simulink model "BLDC_PWM_control"  (R2024b)
settings: Solver=odeN  StartTime=0.0  StopTime=35  MaxStep=Ts_motor  RelTol=1e-3  EnableMultiTasking=on
InitFcn:
  | load bldcData
model workspace (MAT data in the model file):
  encoderResolution = 2000
  hallOffset = '0.5'
  indexOffset = 850
  polePairs = '4'
undefined symbols (not defined in the file): DiscIntNeverNeededParam, Ts_motor
libraries: nesl_utility x14, fl_lib x9, ee_lib x7, spsPWMGeneratorDCDCLib x1, slpidlib x1, simulink x1
settings Model: SimulationMode=accelerator  Creator=The MathWorks, Inc.
settings SolverCC: AlgebraicLoopSolver=TrustRegion  AutoInsertRateTranBlk=on
settings DataIOCC: LimitDataPoints=on  SaveFormat=Array  SaveOutput=off  SaveTime=off  ReturnWorkspaceOutputs=off
settings OptimizationCC: DefaultParameterBehavior=Inlined  OptimizeBlockIOStorage=off  BufferReuse=off  GlobalBufferReuse=off  ExpressionFolding=off  ExpressionDepthLimit=2147483647  LocalBlockOutputs=off  ZeroExternalMemoryAtStartup=off  InitFltsAndDblsToZero=on  NoFixptDivByZeroProtection=on  EfficientFloat2IntCast=on  EfficientMapNaN2IntZero=off  LifeSpan=Inf  MaxStackSize=64  OptimizeDataStoreBuffers=off  BusAssignmentInplaceUpdate=off  EfficientTunableParamExpr=on
settings DebuggingCC: ReadBeforeWriteMsg=DisableAll  WriteAfterWriteMsg=DisableAll  WriteAfterReadMsg=DisableAll  CheckSSInitialOutputMsg=off  SignalResolutionControl=TryResolveAllWithWarning  SolverPrmCheckMsg=warning  InheritedTsInSrcMsg=none  MultiTaskDSMMsg=none  MultiTaskCondExecSysMsg=none  TasksWithSamePriorityMsg=none  SigSpecEnsureSampleTimeMsg=none  IntegerOverflowMsg=none  ParameterPrecisionLossMsg=none  FcnCallInpInsideContextMsg=warning  UnconnectedInputMsg=warning  UnconnectedOutputMsg=warning  UnconnectedLineMsg=warning  AllowSymbolicDim=off  StateNameClashWarn=warning  PregeneratedLibrarySubsystemCodeDiagnostic=none  SFUnexpectedBacktrackingDiag=warning  SFNoUnconditionalDefaultTransitionDiag=warning  SFExecutionAtInitializationDiag=none  IntegerSaturationMsg=none  ArithmeticOperatorsInVariantConditions=warning
settings HardwareCC: ProdBitPerChar=16  ProdBitPerInt=16  ProdBitPerPointer=32  ProdBitPerSizeT=32  ProdBitPerPtrDiffT=32  ProdLargestAtomicInteger=Integer  ProdLargestAtomicFloat=None  ProdWordSize=16  ProdLongLongMode=on  ProdHWDeviceType=Texas Instruments->C2000  TargetBitPerChar=16  TargetBitPerInt=16  TargetBitPerPointer=16  TargetLargestAtomicInteger=Integer  TargetIntDivRoundTo=Zero  TargetEndianess=LittleEndian  TargetWordSize=16  TargetHWDeviceType=TI C2000
settings ModelReferenceCC: EnableRefExpFcnMdlSchedulingChecks=on  PropagateSignalLabelsOutOfModel=off
settings SFSimCC: SimUseLocalCustomCode=off  MATLABDynamicMemAlloc=off
settings RTWCC: Description=Embedded Coder  SystemTargetFile=ert.tlc  TemplateMakefile=ert_default_tmf  GenerateReport=on  RTWUseLocalCustomCode=off  Toolchain=Texas Instruments Code Composer Studio (C2000)  IncludeHyperlinkInReport=on  LaunchReport=on  GenerateTraceInfo=on  GenerateTraceReport=on  GenerateTraceReportSl=on  GenerateTraceReportSf=on  GenerateTraceReportEml=on  GPUComputeCapability=3.5
settings CodeAppCC: IgnoreCustomStorageClasses=off  CustomSymbolStrType=$N$R$M  StateflowObjectComments=on  InternalIdentifier=Classic
settings ERTTargetCC: MultiwordLength=2048  InlinedParameterPlacement=Hierarchical  ERTCustomFileTemplate=example_file_process.tlc  ConvertIfToSwitch=off  SuppressUnreachableDefaultCases=off  MemSecPackage=tic2000demospkg  DynamicArrayContainerType=coder::array
settings ConfigComp: CovMetricSettings=dw  CovSaveCumulativeToWorkspaceVar=on  CovSaveSingleToWorkspaceVar=on  CovExternalEMLEnable=off  CovSFcnEnable=off

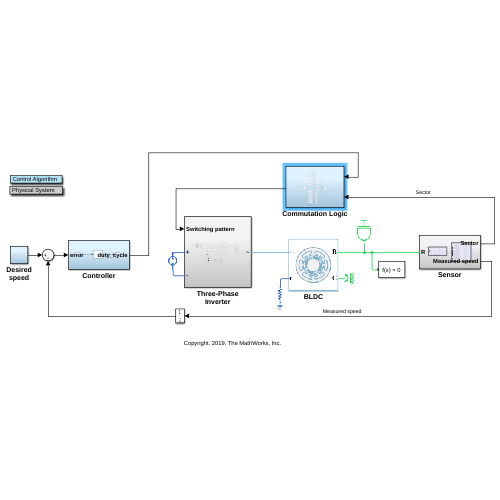
[thumbnail: Simulink's stored preview of the top-level diagram]
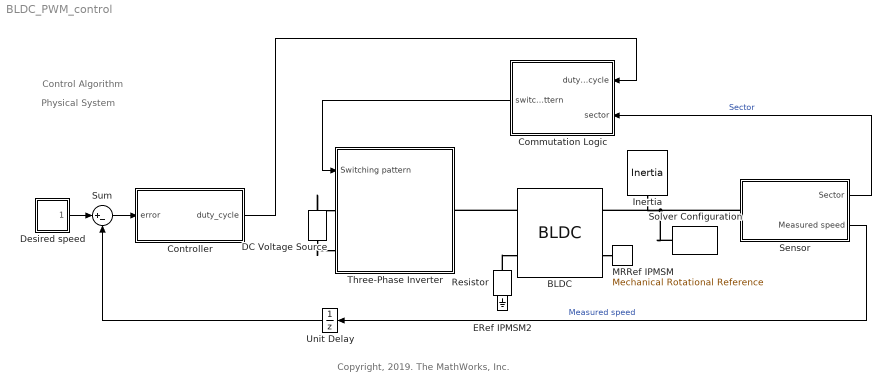
== system BLDC_PWM_control ==
  note: Copyright, 2019. The MathWorks, Inc.
  note: Control Algorithm
  note: Physical System
  BLDC : ee_lib/Electromechanical/Permanent Magnet/BLDC  port_option=ee.enum.threePhasePort.composite  rotor_param=1  pm_flux_linkage=0.18 Wb  theta_constant=120/4 deg  emf_max=9.6 V  w_meas=600 rpm  DphiDtheta_tab=[0, -.1528, -.1528, .1528, .1528, 0] Wb/rad  back_emf_tab=[0, -9.6, -9.6, 9.6, 9.6, 0] V  rotor_angle_tab=[0, 7.5, 22.5, 37.5, 52.5, 60] deg  nPolePairs=4  axes_param=1  winding_type=ee.enum.statorconnection.wye  stator_param=ee.enum.statorparam.LdLqL0  machine_param=ee.enum.dqparameterization.constant  Ld=0.0001 H  Lq=0.0001 H  idVec=[-200, 0, 200] A  iqVec=[-200, 0, 200] A  LdMatrix=0.00022 * ones(3, 3) H  LqMatrix=0.00022 * ones(3, 3) H  L0=0.00016 H  Ls=0.0002 H  Lm=0 H  Ms=0.00002 H  Rs=0.001 Ohm  zero_sequence=ee.enum.park.zerosequence.include  loss_param=ee.enum.ironloss.none  losses_oc=[0, 0, 0] W  losses_sc=[0, 0, 0] W  f_losses=60 Hz  Isc_losses=95 A  J=0 kg*m^2  lam=0.1 N*m/(rad/s)  i_d_specify=off  i_d_priority=None  i_d=0 A  i_d_nominal_specify=off  i_d_nominal_value=1  i_d_nominal_unit=A  i_q_specify=off  i_q_priority=None  i_q=0 A  i_q_nominal_specify=off  i_q_nominal_value=1  i_q_nominal_unit=A  torque_specify=off  torque_priority=None  torque=0 N*m  torque_nominal_specify=off  torque_nominal_value=1  torque_nominal_unit=N*m  angular_velocity_specify=off  angular_velocity_priority=High  angular_velocity=0 rpm  angular_velocity_nominal_specify=off  angular_velocity_nominal_value=1  angular_velocity_nominal_unit=rpm  angular_position_specify=off  angular_position_priority=High  angular_position=0 deg  angular_position_nominal_specify=off  angular_position_nominal_value=1  angular_position_nominal_unit=deg  alpha=3.93e-3 1/K  alpha_flux=-0.001 1/K  Tmeas=298.15 K  stator_thermal_mass=100 J/K  rotor_thermal_mass=200 J/K  Rm_percent_rotor=90  Rd_percent_rotor=30  temperatureA_specify=off  temperatureA_priority=High  temperatureA=25 degC  temperatureA_nominal_specify=off  temperatureA_nominal_value=1  temperatureA_nominal_unit=degC  temperatureB_specify=off  temperatureB_priority=High  temperatureB=25 degC  temperatureB_nominal_specify=off  temperatureB_nominal_value=1  temperatureB_nominal_unit=degC  temperatureC_specify=off  temperatureC_priority=High  temperatureC=25 degC  temperatureC_nominal_specify=off  temperatureC_nominal_value=1  temperatureC_nominal_unit=degC  temperatureR_specify=off  temperatureR_priority=High  temperatureR=25 degC  temperatureR_nominal_specify=off  temperatureR_nominal_value=1  temperatureR_nominal_unit=degC
      settings: InternalSimscapePortConfiguration="{\"Bottom\":[],\"Left\":[{\"id\":\"N\",\"label\":\"~\",\"type\":\"foundation.electrical.three_phase\"},{\"id\":\"n\",\"label\":\"n\",\"type\":\"foundation.electrical.electrical\"}],\"Right\":[{\"id\":\"R\",\"label\":\"R\",\"type\":\"foundation.mechanical.rotational.rotational\"},{\"id\":\"C\",\"label\":\"C\",\"type\":\"foundation.mechanical.rotational.rotational\"}],\"Top\":[]}"
  Commutation Logic : Subsystem
  Controller : Subsystem
  DC Voltage Source : ee_lib/Additional Components/SPICE Sources/DC Voltage Source  DC=500 V
  Desired speed : Subsystem
  ERef IPMSM2 : fl_lib/Electrical/Electrical Elements/Electrical Reference
  Inertia : fl_lib/Mechanical/Rotational Elements/Inertia  inertia=2 kg*m^2  num_ports=foundation.enum.numPorts2.one  w_specify=off  w_priority=High  w=0 rpm  w_nominal_specify=off  w_nominal_value=1  w_nominal_unit=rad/s  t_specify=off  t_priority=High  t=0 N*m  t_nominal_specify=off  t_nominal_value=1  t_nominal_unit=N*m
  MRRef IPMSM : fl_lib/Mechanical/Rotational Elements/Mechanical Rotational Reference
  Resistor : fl_lib/Electrical/Electrical Elements/Resistor  R=1e9 Ohm  i_specify=off  i_priority=None  i=0 A  i_nominal_specify=off  i_nominal_value=1  i_nominal_unit=A  v_specify=off  v_priority=None  v=0 V  v_nominal_specify=off  v_nominal_value=1  v_nominal_unit=V
  Sensor : Subsystem
  Solver Configuration : nesl_utility/Solver Configuration  PhysicalDomain=network_engine_domain  SubClassName=solver  LeftPortType=input  RightPortType=generic  Tones=[]  Harmonics=[]  SimulateNoise=off  Profile=off  UseLocalSampling=off  EnableSwitchedLinearOptims=on  FrequencyDomain=off  UseCCode=off  RelTol=0.001  AbsTol=1e-06  MinStep=1e-09  ToWorkspace=off  RevertToSquareIcSolve=off  NumHomotopyIterations=100  PhasorMode=off  PhasorModeNumHarmonics=1  ConsistencySolver=NEWTON_FTOL  IndexReductionMethod=DerivativeReplacement  DoDC=off  ResidualTolerance=1e-09  ConsistencyTolSource=GLOBAL  ConsistencyAbsTol=0.001  ConsistencyRelTol=0.001  ConsistencyTolFactor=0.001  UseLocalSolver=on  LocalSolverChoice=NE_BACKWARD_EULER_ADVANCER  ResolveIndetEquations=on  FunctionEvalNumThread=1  LocalSolverSampleTime=Ts_motor  DoFixedCost=on  MaxNonlinIter=2  MaxModeIter=2  ComputeImpulses=off  ImpulseIterations=2  LinearAlgebra=auto  LinearAlgebraNumThread=0  EquationFormulation=NE_TIME_EF  DelaysMemoryBudget=1024  AutomaticFiltering=on  FilteringTimeConstant=0.001  PartitionStorageMethod=AS_NEEDED  PartitionMemoryBudget=1024  PartitionMethod=FAST  MultibodyUseLocalSolver=off  MultibodyLocalSolverChoice=ODE1  MultibodyLocalSolverSampleTime=0.001
  Sum : Sum  Inputs=|+-
  Three-Phase Inverter : Subsystem
  Unit Delay : UnitDelay  SampleTime=-1  HasFrameUpgradeWarning=on
  wires:
  Sensor/1(Sector) -> Commutation Logic/2(sector)  "Sector"
  Sum/1 -> Controller/1(error)
  Unit Delay/1 -> Sum/2
  Desired speed/1(Out1) -> Sum/1
  Sensor/2(Measured speed) -> Unit Delay/1  "Measured speed"
  Commutation Logic/1("  switching_pattern") -> Three-Phase Inverter/1(Switching pattern)
  Controller/1(duty_cycle) -> Commutation Logic/1(duty_cycle)
  connections:
  BLDC/RConn2 -- MRRef IPMSM/LConn1
  Sensor/LConn1 -- Inertia/LConn1 -- BLDC/RConn1 -- Solver Configuration/RConn1
  Resistor/LConn1 -- BLDC/LConn2
  ERef IPMSM2/LConn1 -- Resistor/RConn1
  DC Voltage Source/LConn1 -- Three-Phase Inverter/LConn1
  DC Voltage Source/RConn1 -- Three-Phase Inverter/LConn2
  BLDC/LConn1 -- Three-Phase Inverter/RConn1

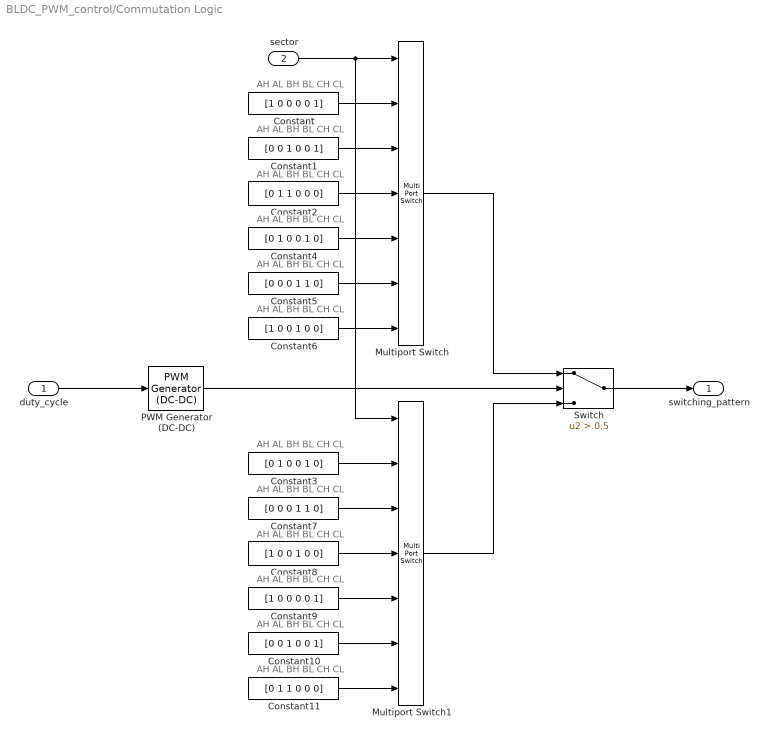
== system BLDC_PWM_control/Commutation Logic ==
  note: AH AL BH BL CH CL
  note: AH AL BH BL CH CL
  note: AH AL BH BL CH CL
  note: AH AL BH BL CH CL
  note: AH AL BH BL CH CL
  note: AH AL BH BL CH CL
  note: AH AL BH BL CH CL
  note: AH AL BH BL CH CL
  note: AH AL BH BL CH CL
  note: AH AL BH BL CH CL
  note: AH AL BH BL CH CL
  note: AH AL BH BL CH CL
  duty_cycle : Inport
  sector : Inport  Port=2
  Constant : Constant  Value=[1 0 0 0 0 1]
  Constant1 : Constant  Value=[0 0 1 0 0 1]
  Constant10 : Constant  Value=[0 0 1 0 0 1]
  Constant11 : Constant  Value=[0 1 1 0 0 0]
  Constant2 : Constant  Value=[0 1 1 0 0 0]
  Constant3 : Constant  Value=[0 1 0 0 1 0]
  Constant4 : Constant  Value=[0 1 0 0 1 0]
  Constant5 : Constant  Value=[0 0 0 1 1 0]
  Constant6 : Constant  Value=[1 0 0 1 0 0]
  Constant7 : Constant  Value=[0 0 0 1 1 0]
  Constant8 : Constant  Value=[1 0 0 1 0 0]
  Constant9 : Constant  Value=[1 0 0 0 0 1]
  Multiport Switch : MultiPortSwitch  Inputs=6  SaturateOnIntegerOverflow=off  InputSameDT=off
  Multiport Switch1 : MultiPortSwitch  Inputs=6  SaturateOnIntegerOverflow=off  InputSameDT=off
  PWM Generator (DC-DC) : spsPWMGeneratorDCDCLib/PWM Generator (DC-DC)  Fsw=1000  Ts=Ts_motor
  Switch : Switch  Criteria=u2 > Threshold  Threshold=0.5  SaturateOnIntegerOverflow=off  InputSameDT=off
  "  switching_pattern" : Outport  VectorParamsAs1DForOutWhenUnconnected=off
  wires:
  Constant6/1 -> Multiport Switch/7
  Constant4/1 -> Multiport Switch/5
  sector/1 -> Multiport Switch1/1, Multiport Switch/1
  Constant1/1 -> Multiport Switch/3
  Constant2/1 -> Multiport Switch/4
  Constant5/1 -> Multiport Switch/6
  Constant/1 -> Multiport Switch/2
  Constant9/1 -> Multiport Switch1/5
  Constant11/1 -> Multiport Switch1/7
  Constant3/1 -> Multiport Switch1/2
  Constant7/1 -> Multiport Switch1/3
  Constant10/1 -> Multiport Switch1/6
  Constant8/1 -> Multiport Switch1/4
  PWM Generator (DC-DC)/1 -> Switch/2
  Switch/1 -> "  switching_pattern"/1
  Multiport Switch/1 -> Switch/1
  Multiport Switch1/1 -> Switch/3
  duty_cycle/1 -> PWM Generator (DC-DC)/1

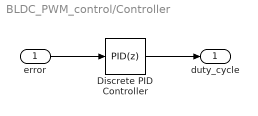
== system BLDC_PWM_control/Controller ==
  error : Inport
  Discrete PID Controller : slpidlib/PID Controller  Controller=PID  Form=Parallel  TimeDomain=Discrete-time  UseExternalTs=off  SampleTime=Ts_motor  IntegratorMethod=Forward Euler  FilterMethod=Forward Euler  ControllerParametersSource=internal  P=0.01  I=0.1  UseKiTs=off  D=0  UseExternalDerivativeSource=off  N=100  UseFilter=on  TunerSelectOption=Transfer Function Based (PID Tuner App)  InitialConditionSource=internal  InitialConditionForIntegrator=0  InitialConditionForFilter=0  DifferentiatorICPrevScaledInput=0  ExternalReset=none  TrackingMode=off  Kt=1  LimitOutput=on  SatLimitsSource=internal  UpperSaturationLimit=1  LowerSaturationLimit=0.5  LinearizeAsGain=off  AntiWindupMode=back-calculation  Kb=1  LimitIntegrator=off  UpperIntegratorSaturationLimit=inf  LowerIntegratorSaturationLimit=-inf  POutMin=[]  POutMax=[]  IOutMin=[]  IOutMax=[]  DOutMin=[]  DOutMax=[]  NOutMin=[]  NOutMax=[]  SumOutMin=[]  SumOutMax=[]  SaturationOutMin=[]  SaturationOutMax=[]  PParamMin=[]  PParamMax=[]  IParamMin=[]  IParamMax=[]  DParamMin=[]  DParamMax=[]  NParamMin=[]  NParamMax=[]  KbParamMin=[]  KbParamMax=[]  KtParamMin=[]  KtParamMax=[]  KbOutMin=[]  KbOutMax=[]  KtOutMin=[]  KtOutMax=[]  IntegratorOutMin=[]  IntegratorOutMax=[]  FilterOutMin=[]  FilterOutMax=[]  SumI1OutMin=[]  SumI1OutMax=[]  SumI2OutMin=[]  SumI2OutMax=[]  SumI3OutMin=[]  SumI3OutMax=[]  SumI4OutMin=[]  SumI4OutMax=[]  SumDOutMin=[]  SumDOutMax=[]  DifferentiatorOutMin=[]  DifferentiatorOutMax=[]  FilterDiffOutCoefMin=[]  FilterDiffOutCoefMax=[]  ReciprocalOutMin=[]  ReciprocalOutMax=[]  SumDenOutMin=[]  SumDenOutMax=[]  SumNumOutMin=[]  SumNumOutMax=[]  DivideOutMin=[]  DivideOutMax=[]  UdiffTsProdOutMin=[]  UdiffTsProdOutMax=[]  NTsProdOutMin=[]  NTsProdOutMax=[]  UintegralTsProdOutMin=[]  UintegralTsProdOutMax=[]  UngainTsProdOutMin=[]  UngainTsProdOutMax=[]  ClampingZeroOutDataTypeStr=Inherit: Inherit via back propagation  ClampingZeroOutMin=[]  ClampingZeroOutMax=[]  FilterDenConstantOutDataTypeStr=Inherit: Inherit via back propagation  FilterDenConstantOutMin=[]  FilterDenConstantOutMax=[]  PCopyOutDataTypeStr=Inherit: Inherit via back propagation  PCopyOutMin=[]  PCopyOutMax=[]  NCopyOutDataTypeStr=Inherit: Inherit via back propagation  NCopyOutMin=[]  NCopyOutMax=[]  IntegratorContinuousStateAttributes=''  IntegratorStateMustResolveToSignalObject=off  IntegratorRTWStateStorageClass=Auto  FilterContinuousStateAttributes=''  FilterStateMustResolveToSignalObject=off  FilterRTWStateStorageClass=Auto  ParallelPVariant=InternalParameters  IdealPVariant=Disabled  IVariant=InternalParameters  DVariant=InternalParameters  IntegratorVariant=Discrete  SatVariant=Enabled  AWVariant=BackCalculation  PCopyVariant=Disabled  TRVariant=Disabled  FdbkBlocksVariant=Forward  IdealPFdbkVariant=Disabled  SatFdbkVariant=Disabled  DerivativeFilterVariant=ForwardEulerFilter  NVariant=InternalParameters  NCopyVariant=Disabled  FilterICVariant=InternalICsFilter  IntegratorICVariant=InternalICs  ExternalResetVariant=Disabled  TRSumVariant=Passthrough  SumFdbkVariant=Disabled  SumVariant=Sum_PID  TsampFilterVariant=InternalTs  TsampNgainVariant=Passthrough  TsampIntegralVariant=Disabled_SignalSpec  ExternalSaturationOutDataTypeStr=Inherit: Same as second input  DerivativeSourceVariant=ErrorSignal  PreIntVariant=InternalPreInt
  duty_cycle : Outport
  wires:
  Discrete PID Controller/1 -> duty_cycle/1
  error/1 -> Discrete PID Controller/1

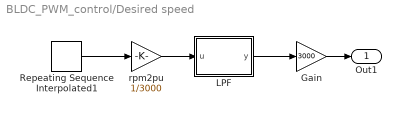
== system BLDC_PWM_control/Desired speed ==
  Gain : Gain  Gain=3000
  LPF : Subsystem
  Repeating Sequence Interpolated1 : simulink/Sources/Repeating Sequence Interpolated  OutValues=[0 1025/2 1025/2 1025 1025 2050 2050 2050]  TimeValues=[0 10 20 30 40 50 60 70]/2  LookUpMeth=Interpolation-Use End Values  tsamp=Ts_motor  OutMin=[]  OutMax=[]  OutDataTypeStr=double  OutputDataTypeScalingMode=double  OutDataType=fixdt(0,8)  OutScaling=2^-10
  rpm2pu : Gain  Gain=1/3000  RndMeth=Simplest  OutDataTypeStr=Inherit: Same as input
  Out1 : Outport
  wires:
  rpm2pu/1 -> LPF/1(u)
  Repeating Sequence Interpolated1/1 -> rpm2pu/1
  LPF/1(y) -> Gain/1
  Gain/1 -> Out1/1

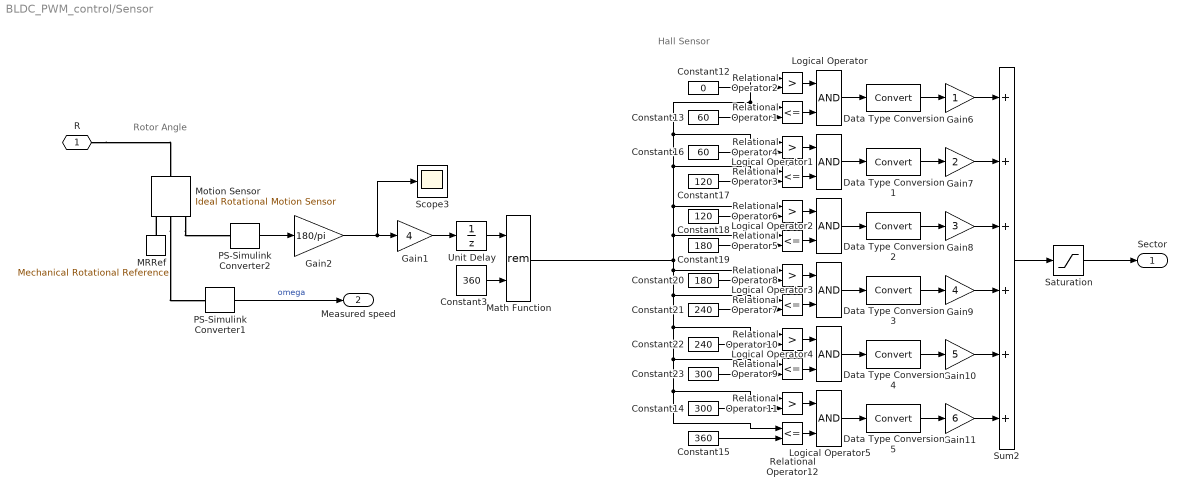
== system BLDC_PWM_control/Sensor ==
  note: Rotor Angle
  note: Hall Sensor
  Constant12 : Constant  Value=0
  Constant13 : Constant  Value=60
  Constant14 : Constant  Value=300
  Constant15 : Constant  Value=360
  Constant16 : Constant  Value=60
  Constant17 : Constant  Value=120
  Constant18 : Constant  Value=120
  Constant19 : Constant  Value=180
  Constant20 : Constant  Value=180
  Constant21 : Constant  Value=240
  Constant22 : Constant  Value=240
  Constant23 : Constant  Value=300
  Constant3 : Constant  Value=360
  Data Type Conversion{,1..5} (6 alike) : DataTypeConversion
  Gain1 : Gain  Gain=4
  Gain10 : Gain  Gain=5  SaturateOnIntegerOverflow=on  OutDataTypeStr=Inherit: Same as input  ParamDataTypeStr=Inherit: Same as input
  Gain11 : Gain  Gain=6  SaturateOnIntegerOverflow=on  OutDataTypeStr=Inherit: Same as input  ParamDataTypeStr=Inherit: Same as input
  Gain2 : Gain  Gain=180/pi
  Gain6 : Gain  SaturateOnIntegerOverflow=on  OutDataTypeStr=Inherit: Same as input  ParamDataTypeStr=Inherit: Same as input
  Gain7 : Gain  Gain=2  SaturateOnIntegerOverflow=on  OutDataTypeStr=Inherit: Same as input  ParamDataTypeStr=Inherit: Same as input
  Gain8 : Gain  Gain=3  SaturateOnIntegerOverflow=on  OutDataTypeStr=Inherit: Same as input  ParamDataTypeStr=Inherit: Same as input
  Gain9 : Gain  Gain=4  SaturateOnIntegerOverflow=on  OutDataTypeStr=Inherit: Same as input  ParamDataTypeStr=Inherit: Same as input
  Logical Operator{,1..5} (6 alike) : Logic
  MRRef : fl_lib/Mechanical/Rotational Elements/Mechanical Rotational Reference
  Math Function : Math  Operator=rem  SignedPower=on
  Motion Sensor : fl_lib/Mechanical/Mechanical Sensors/Ideal Rotational Motion Sensor  reference=foundation.enum.MeasurementReference.difference  acceleration_port=false  velocity_port=true  position_port=true  wrap_angle=false  offset=0 deg
  PS-Simulink Converter1 : nesl_utility/PS-Simulink Converter  PhysicalDomain=network_engine_domain  SubClassName=ps_output  LeftPortType=input  RightPortType=output  PseudoPeriodic=off  Frequencies=[]  VectorFormat=1-D array  Unit=rpm  AffineConversion=off
  PS-Simulink Converter2 : nesl_utility/PS-Simulink Converter  PhysicalDomain=network_engine_domain  SubClassName=ps_output  LeftPortType=input  RightPortType=output  PseudoPeriodic=off  Frequencies=[]  VectorFormat=1-D array  Unit=rad  AffineConversion=off
  Relational Operator{1,3,5,7,9,12} (6 alike) : RelationalOperator  Operator=<=
  Relational Operator{2,4,6,8,10..11} (6 alike) : RelationalOperator  Operator=>
  Saturation : Saturate  UpperLimit=6  LowerLimit=1
  Scope3 : Scope
  Sum2 : Sum  Inputs=++++++  InputSameDT=on  SaturateOnIntegerOverflow=on  OutDataTypeStr=Inherit: Same as first input
  Unit Delay : UnitDelay  SampleTime=Ts_motor  HasFrameUpgradeWarning=on
  R : PMIOPort  Side=Left
  Sector : Outport
  Measured speed : Outport  Port=2
  wires:
  Saturation/1 -> Sector/1
  Math Function/1 -> Relational Operator2/1, Relational Operator1/1, Relational Operator4/1, Relational Operator3/1, Relational Operator6/1, Relational Operator5/1, Relational Operator12/1, Relational Operator11/1, Relational Operator9/1, Relational Operator10/1, Relational Operator7/1, Relational Operator8/1
  Data Type Conversion5/1 -> Gain11/1
  Data Type Conversion4/1 -> Gain10/1
  Data Type Conversion3/1 -> Gain9/1
  Data Type Conversion2/1 -> Gain8/1
  Data Type Conversion1/1 -> Gain7/1
  Data Type Conversion/1 -> Gain6/1
  Relational Operator2/1 -> Logical Operator/1
  Relational Operator1/1 -> Logical Operator/2
  Logical Operator/1 -> Data Type Conversion/1
  Constant12/1 -> Relational Operator2/2
  Constant13/1 -> Relational Operator1/2
  Relational Operator4/1 -> Logical Operator1/1
  Relational Operator3/1 -> Logical Operator1/2
  Logical Operator1/1 -> Data Type Conversion1/1
  Constant16/1 -> Relational Operator4/2
  Constant17/1 -> Relational Operator3/2
  Relational Operator6/1 -> Logical Operator2/1
  Relational Operator5/1 -> Logical Operator2/2
  Logical Operator2/1 -> Data Type Conversion2/1
  Constant18/1 -> Relational Operator6/2
  Constant19/1 -> Relational Operator5/2
  Relational Operator8/1 -> Logical Operator3/1
  Relational Operator7/1 -> Logical Operator3/2
  Logical Operator3/1 -> Data Type Conversion3/1
  Constant20/1 -> Relational Operator8/2
  Constant21/1 -> Relational Operator7/2
  Relational Operator10/1 -> Logical Operator4/1
  Relational Operator9/1 -> Logical Operator4/2
  Logical Operator4/1 -> Data Type Conversion4/1
  Constant22/1 -> Relational Operator10/2
  Constant23/1 -> Relational Operator9/2
  Relational Operator11/1 -> Logical Operator5/1
  Relational Operator12/1 -> Logical Operator5/2
  Logical Operator5/1 -> Data Type Conversion5/1
  Constant14/1 -> Relational Operator11/2
  Constant15/1 -> Relational Operator12/2
  Gain6/1 -> Sum2/1
  Gain7/1 -> Sum2/2
  Gain8/1 -> Sum2/3
  Gain9/1 -> Sum2/4
  Gain10/1 -> Sum2/5
  Gain11/1 -> Sum2/6
  Sum2/1 -> Saturation/1
  PS-Simulink Converter2/1 -> Gain2/1
  Gain2/1 -> Scope3/1, Gain1/1
  Constant3/1 -> Math Function/2
  Gain1/1 -> Unit Delay/1
  Unit Delay/1 -> Math Function/1
  PS-Simulink Converter1/1 -> Measured speed/1  "omega"
  connections:
  Motion Sensor/RConn3 -- PS-Simulink Converter2/LConn1
  MRRef/LConn1 -- Motion Sensor/RConn1
  Motion Sensor/RConn2 -- PS-Simulink Converter1/LConn1
  R/RConn1 -- Motion Sensor/LConn1

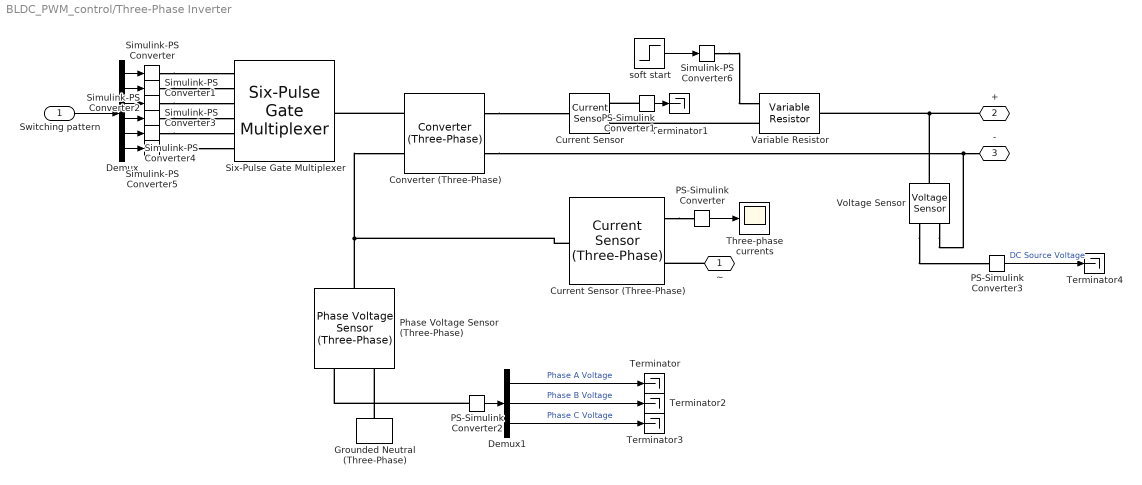
== system BLDC_PWM_control/Three-Phase Inverter ==
  Switching pattern : Inport
  Converter (Three-Phase) : ee_lib/Semiconductors & Converters/Converters/Converter (Three-Phase)  port_option=ee.enum.threePhasePort.composite  fidelity_option=ee.enum.converters.fidelity.detailed  device_type=ee.enum.converters.switchingdevice.ideal  showThermalPort=false  K=0  Vth=0.5 V  Vgt=1 V  Vgt_off=-1 V  Ih=1 A  Vf=0.8 V  Ron=0.001 Ohm  Rds=0.001 Ohm  Goff=0.001 1/Ohm  Eon_scalar=22.86e-3 J  Eoff_scalar=17.14e-3 J  Eoff_natural_commutation=10e-3 J  Voff=300 V  Iout_scalar=600 A  onCurrentMeasDelay=0 s  useCurrentFromPreviousCycle=false  useVoltageFromPreviousCycle=false  diode_param=ee.enum.converters.protectiondiode.nodynamics  diode_Vf=0.8 V  diode_Ron=0.001 Ohm  diode_Goff=1e-5 1/Ohm  diode_C=50 nF  diode_iRM=-235 A  diode_iF=300 A  diode_idot=-50 A/us  diode_trr_param=ee.enum.converters.diodetrr.trr_factor  diode_trr_factor=3  diode_trr=15 us  diode_Qrr=1500 s*uA  diode_rec_loss_model=ee.enum.diode.reverseRecoveryModel.fixed  diode_ErecVal=0 J  diode_scaleWithIandV=false  diode_ErecMat=zeros(2, 3) J  diode_TjrecVec=[298.15, 398.15] K  diode_IfrecVec=[.1, 1, 10] A  diode_IrecVal=10 A  diode_VrecVal=10 V  diode_tFilter=1 / 1000 / 100 s  thermal_network_parameterization=ee.enum.thermalNetworkTopology.external  Rth=[.08, .5] K/W  Rth_Cauer=[.08, .1, .5] K/W  Rth_Foster=[.08, .14, .22, .16] K/W  thermal_mass_parameterization=ee.enum.thermalNetwork.timeconstant  thermal_mass=[.01, .5] J/K  thermal_mass_Cauer=[.01, .1, .5] J/K  thermal_mass_Foster=[.001, .005, .05, .5] J/K  thermal_time_constant=[.001, .2] s  thermal_time_constant_Cauer=[.001, .1, .2] s  thermal_time_constant_Foster=[7e-05, .0007, .01, .08] s  thermal_mass_initial_temperatures=[25, 25] degC  thermal_mass_initial_temperatures_Cauer=[25, 25, 25] degC  junction_thermal_mass=0.01 J/K  Tvec_initial_Foster=[25, 25, 25, 25] degC  snubber_type=ee.enum.converters.snubber.exclude  Cs=1e-7 F  Rs=0.1 Ohm  Vce_loss=[0, 150, 300] V
  Current Sensor : fl_lib/Electrical/Electrical Sensors/Current Sensor
  Current Sensor (Three-Phase) : ee_lib/Sensors & Transducers/Current Sensor (Three-Phase)
  Demux : Demux  Outputs=6
  Demux1 : Demux  Outputs=3
  Grounded Neutral (Three-Phase) : ee_lib/Connectors & References/Grounded Neutral (Three-Phase)
  PS-Simulink Converter : nesl_utility/PS-Simulink Converter  PhysicalDomain=network_engine_domain  SubClassName=ps_output  LeftPortType=input  RightPortType=output  PseudoPeriodic=off  Frequencies=[]  VectorFormat=1-D array  Unit=1  AffineConversion=off
  PS-Simulink Converter1 : nesl_utility/PS-Simulink Converter  PhysicalDomain=network_engine_domain  SubClassName=ps_output  LeftPortType=input  RightPortType=output  PseudoPeriodic=off  Frequencies=[]  VectorFormat=1-D array  Unit=inherit  AffineConversion=off
  PS-Simulink Converter2 : nesl_utility/PS-Simulink Converter  PhysicalDomain=network_engine_domain  SubClassName=ps_output  LeftPortType=input  RightPortType=output  PseudoPeriodic=off  Frequencies=[]  VectorFormat=1-D array  Unit=inherit  AffineConversion=off
  PS-Simulink Converter3 : nesl_utility/PS-Simulink Converter  PhysicalDomain=network_engine_domain  SubClassName=ps_output  LeftPortType=input  RightPortType=output  PseudoPeriodic=off  Frequencies=[]  VectorFormat=1-D array  Unit=inherit  AffineConversion=off
  Phase Voltage Sensor (Three-Phase) : ee_lib/Sensors & Transducers/Phase Voltage Sensor (Three-Phase)
  Simulink-PS Converter{,1..6} (7 alike) : nesl_utility/Simulink-PS Converter  PhysicalDomain=network_engine_domain  SubClassName=ps_input  LeftPortType=input  RightPortType=output  PseudoPeriodic=off  Frequencies=[]  NoiseDistribution=none  NoiseParameters=[]  Unit=1  AffineConversion=off  FilteringAndDerivatives=provide  SimscapeFilterOrder=1  InputFilterTimeConstant=0.001  UdotUserProvided=0
  Six-Pulse Gate Multiplexer : ee_lib/Semiconductors & Converters/Converters/Six-Pulse Gate Multiplexer  port_option=ee.enum.controlport.ps
  Terminator{,1..4} (5 alike) : Terminator
  Three-phase currents : Scope
  Variable Resistor : fl_lib/Electrical/Electrical Elements/Variable Resistor  Rmin=0 Ohm  thermalEnable=false  thermal_mass=1 J/K  i_specify=off  i_priority=None  i=0 A  i_nominal_specify=off  i_nominal_value=1  i_nominal_unit=A  v_specify=off  v_priority=None  v=0 V  v_nominal_specify=off  v_nominal_value=1  v_nominal_unit=V  T_specify=off  T_priority=None  T=300 K  T_nominal_specify=off  T_nominal_value=1  T_nominal_unit=K
  Voltage Sensor : fl_lib/Electrical/Electrical Sensors/Voltage Sensor
  soft start : Step  Time=4  Before=0.5  After=1e-3  SampleTime=Ts_motor
  ~ : PMIOPort  Side=Right
  + : PMIOPort  Port=2  Side=Left
  - : PMIOPort  Port=3  Side=Left
  wires:
  PS-Simulink Converter/1 -> Three-phase currents/1
  Switching pattern/1 -> Demux/1
  Demux/1 -> Simulink-PS Converter/1
  Demux/2 -> Simulink-PS Converter1/1
  Demux/3 -> Simulink-PS Converter2/1
  Demux/4 -> Simulink-PS Converter3/1
  Demux/5 -> Simulink-PS Converter4/1
  Demux/6 -> Simulink-PS Converter5/1
  PS-Simulink Converter2/1 -> Demux1/1
  soft start/1 -> Simulink-PS Converter6/1
  PS-Simulink Converter1/1 -> Terminator1/1
  Demux1/1 -> Terminator/1  "Phase A Voltage"
  Demux1/2 -> Terminator2/1  "Phase B Voltage"
  Demux1/3 -> Terminator3/1  "Phase C Voltage"
  PS-Simulink Converter3/1 -> Terminator4/1  "DC Source Voltage"
  connections:
  Current Sensor (Three-Phase)/RConn1 -- PS-Simulink Converter/LConn1
  Simulink-PS Converter/RConn1 -- Six-Pulse Gate Multiplexer/LConn1
  Simulink-PS Converter1/RConn1 -- Six-Pulse Gate Multiplexer/LConn2
  Simulink-PS Converter2/RConn1 -- Six-Pulse Gate Multiplexer/LConn3
  Simulink-PS Converter3/RConn1 -- Six-Pulse Gate Multiplexer/LConn4
  Simulink-PS Converter4/RConn1 -- Six-Pulse Gate Multiplexer/LConn5
  Simulink-PS Converter5/RConn1 -- Six-Pulse Gate Multiplexer/LConn6
  Converter (Three-Phase)/LConn1 -- Six-Pulse Gate Multiplexer/RConn1
  Converter (Three-Phase)/RConn1 -- Current Sensor/LConn1
  Converter (Three-Phase)/RConn2 -- Voltage Sensor/RConn2 -- -/RConn1
  Current Sensor (Three-Phase)/LConn1 -- Converter (Three-Phase)/LConn2 -- Phase Voltage Sensor (Three-Phase)/LConn1
  ~/RConn1 -- Current Sensor (Three-Phase)/RConn2
  Grounded Neutral (Three-Phase)/LConn1 -- Phase Voltage Sensor (Three-Phase)/RConn2
  PS-Simulink Converter2/LConn1 -- Phase Voltage Sensor (Three-Phase)/RConn1
  PS-Simulink Converter1/LConn1 -- Current Sensor/RConn1
  Variable Resistor/LConn2 -- Current Sensor/RConn2
  +/RConn1 -- Voltage Sensor/LConn1 -- Variable Resistor/RConn1
  Simulink-PS Converter6/RConn1 -- Variable Resistor/LConn1
  Voltage Sensor/RConn1 -- PS-Simulink Converter3/LConn1

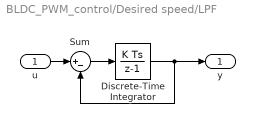
== system BLDC_PWM_control/Desired speed/LPF ==
  u : Inport
  Discrete-Time Integrator : DiscreteIntegrator  gainval=20  SampleTime=Ts_motor  ICPrevOutput=DiscIntNeverNeededParam  ICPrevScaledInput=DiscIntNeverNeededParam
  Sum : Sum  Inputs=|+-
  y : Outport
  wires:
  Sum/1 -> Discrete-Time Integrator/1
  Discrete-Time Integrator/1 -> y/1, Sum/2
  u/1 -> Sum/1
